simulink model "CSAD_DWC3_linear_4corner"  (R2017a)
settings: Solver=ode5  StartTime=0.0  StopTime=t_sim  FixedStep=0.01  MaxStep=0.01  RelTol=1e-3
values from neighbouring files (symbols this model uses):
  eta_initial = [5; -1; 0]    [Run4corner.m]    (also in Simulation_plot.m = [-4; -2; 0.6*pi])
  nu_initial = [0; 0; 0]    [Run4corner.m]    (also in Simulation_plot.m)
settings Model: Creator=ONLyn  LastModifiedBy=ONLyn

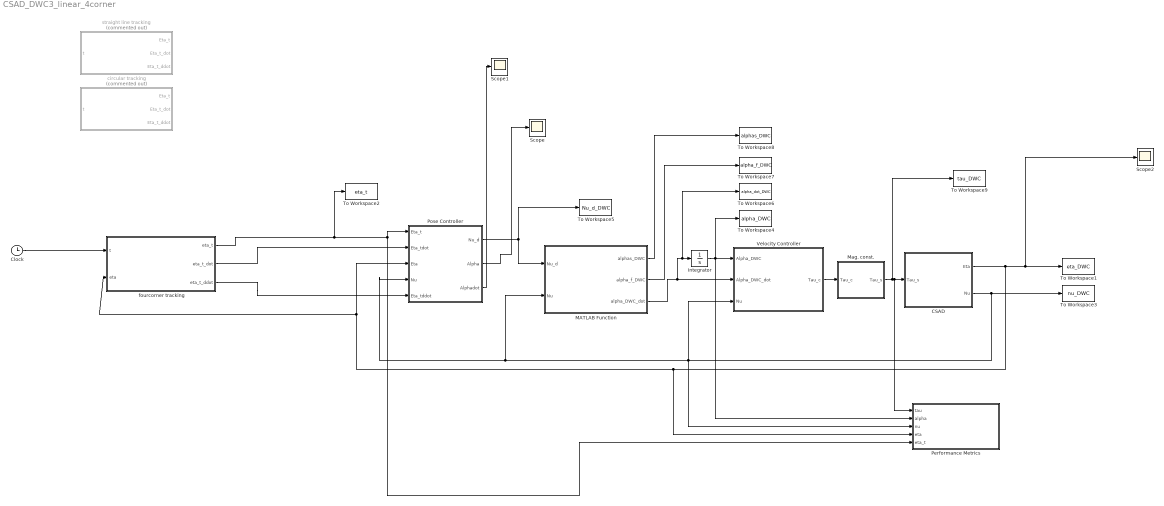
== system CSAD_DWC3_linear_4corner ==
  " Pose Controller" : MATLAB Function  TreatAsAtomicUnit=on
  " Velocity Controller" : MATLAB Function  TreatAsAtomicUnit=on
  " straight line tracking" : MATLAB Function  Commented=on  TreatAsAtomicUnit=on
  CSAD : Subsystem
  Clock : Clock
  Integrator : Integrator  InitialCondition=[0 0 0]
  MATLAB Function : MATLAB Function  TreatAsAtomicUnit=on
  Mag. const. : MATLAB Function  TreatAsAtomicUnit=on
  "Performance Metrics " : Subsystem
  Scope : Scope
  Scope1 : Scope
  Scope2 : Scope
  To Workspace1 : ToWorkspace  VariableName=eta_DWC  SampleTime=-1
  To Workspace2 : ToWorkspace  VariableName=eta_t  SampleTime=-1
  To Workspace3 : ToWorkspace  VariableName=nu_DWC  SampleTime=-1
  To Workspace4 : ToWorkspace  VariableName=alpha_DWC  SampleTime=-1
  To Workspace5 : ToWorkspace  VariableName=Nu_d_DWC  SampleTime=-1
  To Workspace6 : ToWorkspace  VariableName=alpha_dot_DWC  SampleTime=-1
  To Workspace7 : ToWorkspace  VariableName=alpha_f_DWC  SampleTime=-1
  To Workspace8 : ToWorkspace  VariableName=alphas_DWC  SampleTime=-1
  To Workspace9 : ToWorkspace  VariableName=tau_DWC  SampleTime=-1
  circular tracking : MATLAB Function  Commented=on  TreatAsAtomicUnit=on
  fourcorner tracking : Subsystem
  wires:
  CSAD/2(Nu) -> To Workspace3/1, "Performance Metrics "/3(nu), " Velocity Controller"/3(Nu), MATLAB Function/2(Nu), " Pose Controller"/4(Nu)
  CSAD/1(Eta) -> Scope2/1, To Workspace1/1, "Performance Metrics "/4(eta), fourcorner tracking/2(eta), " Pose Controller"/3(Eta)
  " Pose Controller"/1(Nu_d) -> To Workspace5/1, MATLAB Function/1(Nu_d)
  Integrator/1 -> " Velocity Controller"/1(Alpha_DWC), To Workspace4/1, "Performance Metrics "/2(alpha)
  Mag. const./1(Tau_s) -> To Workspace9/1, "Performance Metrics "/1(tau), CSAD/1(Tau_s)
  MATLAB Function/3(alpha_DWC_dot) -> " Velocity Controller"/2(Alpha_DWC_dot), To Workspace6/1, Integrator/1
  MATLAB Function/2(alpha_f_DWC) -> To Workspace7/1
  MATLAB Function/1(alphas_DWC) -> To Workspace8/1
  " Velocity Controller"/1(Tau_c) -> Mag. const./1(Tau_c)
  " Pose Controller"/2(Alpha) -> Scope/1
  " Pose Controller"/3(Alphadot) -> Scope1/1
  fourcorner tracking/1(eta_t) -> "Performance Metrics "/5(eta_t), " Pose Controller"/1(Eta_t), To Workspace2/1
  Clock/1 -> fourcorner tracking/1(t)
  fourcorner tracking/2(eta_t_dot) -> " Pose Controller"/2(Eta_tdot)
  fourcorner tracking/3(eta_t_ddot) -> " Pose Controller"/5(Eta_tddot)

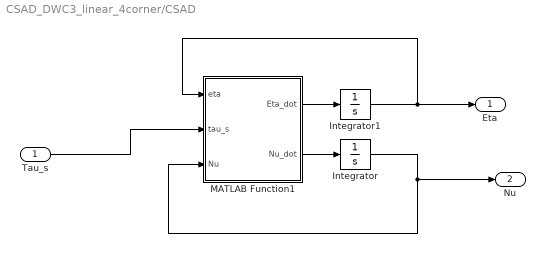
== system CSAD_DWC3_linear_4corner/CSAD ==
  Tau_s : Inport
  Integrator : Integrator  InitialCondition=nu_initial
  Integrator1 : Integrator  InitialCondition=eta_initial
  MATLAB Function1 : MATLAB Function  TreatAsAtomicUnit=on
  Eta : Outport
  Nu : Outport  Port=2
  wires:
  Integrator/1 -> Nu/1, MATLAB Function1/3(Nu)
  MATLAB Function1/1(Eta_dot) -> Integrator1/1
  Integrator1/1 -> Eta/1, MATLAB Function1/1(eta)
  MATLAB Function1/2(Nu_dot) -> Integrator/1
  Tau_s/1 -> MATLAB Function1/2(tau_s)

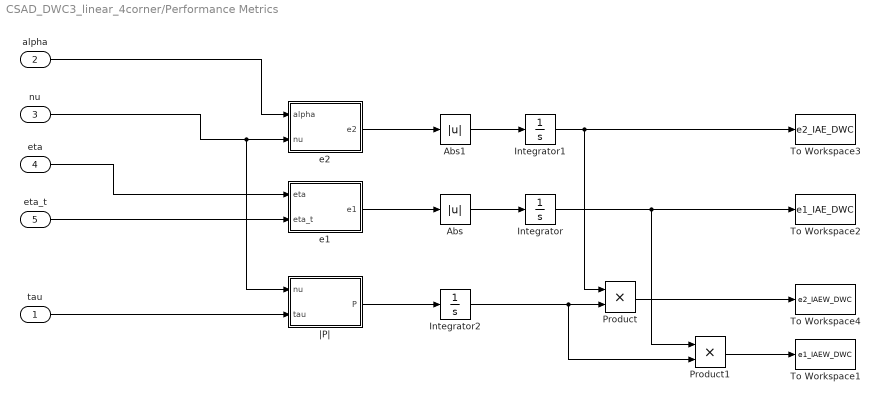
== system CSAD_DWC3_linear_4corner/Performance Metrics  ==
  tau : Inport
  alpha : Inport  Port=2
  nu : Inport  Port=3
  eta : Inport  Port=4
  eta_t : Inport  Port=5
  Abs : Abs
  Abs1 : Abs
  Integrator : Integrator
  Integrator1 : Integrator
  Integrator2 : Integrator
  Product : Product
  Product1 : Product
  To Workspace1 : ToWorkspace  VariableName=e1_IAEW_DWC  SampleTime=-1
  To Workspace2 : ToWorkspace  VariableName=e1_IAE_DWC  SampleTime=-1
  To Workspace3 : ToWorkspace  VariableName=e2_IAE_DWC  SampleTime=-1
  To Workspace4 : ToWorkspace  VariableName=e2_IAEW_DWC  SampleTime=-1
  e1 : MATLAB Function  TreatAsAtomicUnit=on
  "e2 " : MATLAB Function  TreatAsAtomicUnit=on
  |P| : MATLAB Function  TreatAsAtomicUnit=on
  wires:
  Integrator/1 -> Product1/1, To Workspace2/1
  e1/1(e1) -> Abs/1
  "e2 "/1(e2) -> Abs1/1
  Integrator1/1 -> Product/1, To Workspace3/1
  Abs/1 -> Integrator/1
  Abs1/1 -> Integrator1/1
  eta_t/1 -> e1/2(eta_t)
  eta/1 -> e1/1(eta)
  nu/1 -> |P|/1(nu), "e2 "/2(nu)
  alpha/1 -> "e2 "/1(alpha)
  tau/1 -> |P|/2(tau)
  |P|/1(P) -> Integrator2/1
  Integrator2/1 -> Product1/2, Product/2
  Product/1 -> To Workspace4/1
  Product1/1 -> To Workspace1/1

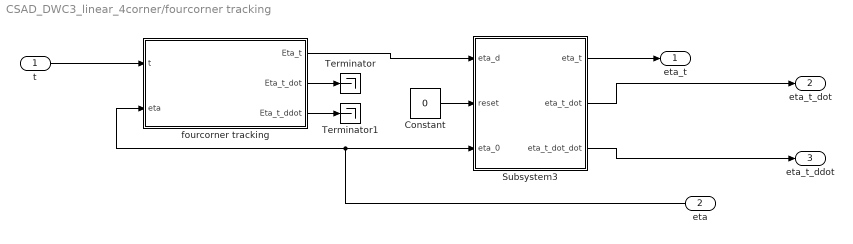
== system CSAD_DWC3_linear_4corner/fourcorner tracking ==
  t : Inport
  eta : Inport  Port=2
  Constant : Constant  Value=0
  Subsystem3 : Subsystem
  Terminator : Terminator
  Terminator1 : Terminator
  fourcorner tracking : MATLAB Function  TreatAsAtomicUnit=on
  eta_t : Outport
  eta_t_dot : Outport  Port=2
  eta_t_ddot : Outport  Port=3
  wires:
  Subsystem3/3(eta_t_dot_dot) -> eta_t_ddot/1
  fourcorner tracking/2(Eta_t_dot) -> Terminator/1
  Constant/1 -> Subsystem3/2(reset)
  Subsystem3/1(eta_t) -> eta_t/1
  t/1 -> fourcorner tracking/1(t)
  eta/1 -> fourcorner tracking/2(eta), Subsystem3/3(eta_0)
  fourcorner tracking/3(Eta_t_ddot) -> Terminator1/1
  fourcorner tracking/1(Eta_t) -> Subsystem3/1(eta_d)
  Subsystem3/2(eta_t_dot) -> eta_t_dot/1

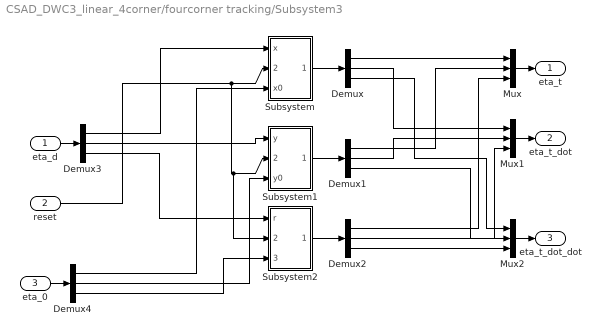
== system CSAD_DWC3_linear_4corner/fourcorner tracking/Subsystem3 ==
  eta_d : Inport
  reset : Inport  Port=2
  eta_0 : Inport  Port=3
  Demux{,1..4} (5 alike) : Demux  Outputs=3
  Mux : Mux  Inputs=3
  Mux1 : Mux  Inputs=3
  Mux2 : Mux  Inputs=3
  Subsystem : Subsystem
  Subsystem1 : Subsystem
  Subsystem2 : Subsystem
  eta_t : Outport  PortDimensions=3
  eta_t_dot : Outport  Port=2  PortDimensions=3
  eta_t_dot_dot : Outport  Port=3  PortDimensions=3
  wires:
  Subsystem1/1(y,yd,ydd) -> Demux1/1
  Subsystem2/1(y,yd,ydd) -> Demux2/1
  Subsystem/1(x,xd,xdd) -> Demux/1
  Demux/3 -> Mux2/1
  eta_d/1 -> Demux3/1
  Mux1/1 -> eta_t_dot/1
  Demux/1 -> Mux/1
  Mux2/1 -> eta_t_dot_dot/1
  Demux3/1 -> Subsystem/1(x)
  Demux1/3 -> Mux2/2
  Demux2/3 -> Mux2/3
  Demux1/1 -> Mux/2
  Demux3/2 -> Subsystem1/1(y)
  Demux3/3 -> Subsystem2/1(r)
  Demux2/2 -> Mux1/3
  Demux1/2 -> Mux1/2
  reset/1 -> Subsystem2/2(reset), Subsystem1/2(reset), Subsystem/2(reset)
  Mux/1 -> eta_t/1
  Demux/2 -> Mux1/1
  Demux2/1 -> Mux/3
  Demux4/3 -> Subsystem2/3(psi0)
  Demux4/2 -> Subsystem1/3(y0)
  Demux4/1 -> Subsystem/3(x0)
  eta_0/1 -> Demux4/1

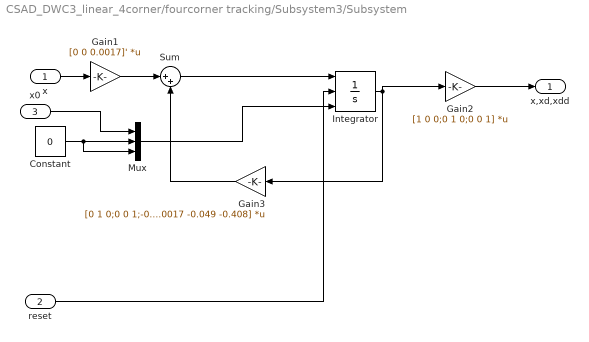
== system CSAD_DWC3_linear_4corner/fourcorner tracking/Subsystem3/Subsystem ==
  x : Inport
  reset : Inport  Port=2
  x0 : Inport  Port=3
  Constant : Constant  Value=0
  Gain1 : Gain  Gain=[0 0 0.0017]'  Multiplication=Matrix(K*u)
  Gain2 : Gain  Gain=[1 0 0;0 1 0;0 0 1]  Multiplication=Matrix(K*u)
  Gain3 : Gain  Gain=[0 1 0;0 0 1;-0.0017 -0.049 -0.408]  Multiplication=Matrix(K*u)
  Integrator : Integrator  ExternalReset=either  InitialConditionSource=external
  Mux : Mux  Inputs=3
  Sum : Sum  Inputs=|++
  x,xd,xdd : Outport  PortDimensions=3
  wires:
  Gain1/1 -> Sum/1
  x/1 -> Gain1/1
  Integrator/1 -> Gain2/1, Gain3/1
  Sum/1 -> Integrator/1
  Gain2/1 -> x,xd,xdd/1
  Mux/1 -> Integrator/3
  reset/1 -> Integrator/2
  Gain3/1 -> Sum/2
  Constant/1 -> Mux/2, Mux/3
  x0/1 -> Mux/1

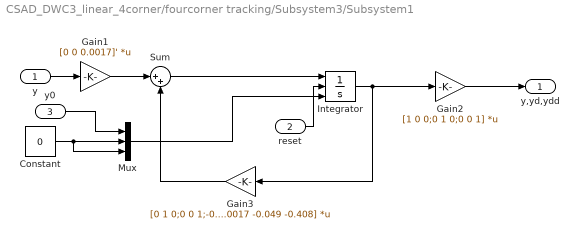
== system CSAD_DWC3_linear_4corner/fourcorner tracking/Subsystem3/Subsystem1 ==
  y : Inport
  reset : Inport  Port=2
  y0 : Inport  Port=3
  Constant : Constant  Value=0
  Gain1 : Gain  Gain=[0 0 0.0017]'  Multiplication=Matrix(K*u)
  Gain2 : Gain  Gain=[1 0 0;0 1 0;0 0 1]  Multiplication=Matrix(K*u)
  Gain3 : Gain  Gain=[0 1 0;0 0 1;-0.0017 -0.049 -0.408]  Multiplication=Matrix(K*u)
  Integrator : Integrator  ExternalReset=either  InitialConditionSource=external
  Mux : Mux  Inputs=3
  Sum : Sum  Inputs=|++
  y,yd,ydd : Outport
  wires:
  Constant/1 -> Mux/3, Mux/2
  Gain3/1 -> Sum/2
  reset/1 -> Integrator/2
  Mux/1 -> Integrator/3
  Gain2/1 -> y,yd,ydd/1
  Sum/1 -> Integrator/1
  Integrator/1 -> Gain3/1, Gain2/1
  y/1 -> Gain1/1
  Gain1/1 -> Sum/1
  y0/1 -> Mux/1

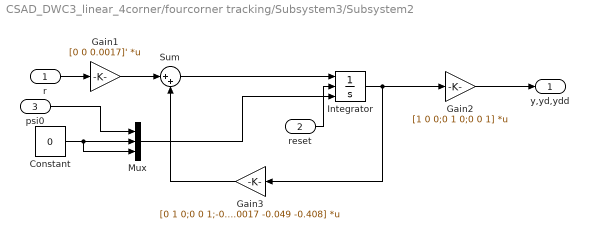
== system CSAD_DWC3_linear_4corner/fourcorner tracking/Subsystem3/Subsystem2 ==
  r : Inport
  reset : Inport  Port=2
  psi0 : Inport  Port=3
  Constant : Constant  Value=0
  Gain1 : Gain  Gain=[0 0 0.0017]'  Multiplication=Matrix(K*u)
  Gain2 : Gain  Gain=[1 0 0;0 1 0;0 0 1]  Multiplication=Matrix(K*u)
  Gain3 : Gain  Gain=[0 1 0;0 0 1;-0.0017 -0.049 -0.408]  Multiplication=Matrix(K*u)
  Integrator : Integrator  ExternalReset=either  InitialConditionSource=external
  Mux : Mux  Inputs=3
  Sum : Sum  Inputs=|++
  y,yd,ydd : Outport
  wires:
  Gain1/1 -> Sum/1
  r/1 -> Gain1/1
  Integrator/1 -> Gain2/1, Gain3/1
  Sum/1 -> Integrator/1
  Gain2/1 -> y,yd,ydd/1
  Mux/1 -> Integrator/3
  reset/1 -> Integrator/2
  Gain3/1 -> Sum/2
  Constant/1 -> Mux/2, Mux/3
  psi0/1 -> Mux/1

== matlab function CSAD_DWC3_linear_4corner/ Velocity Controller ==
  data: Alpha_DWC input; Alpha_DWC_dot input; Tau_c output; Nu input
function Tau_c = VelocityControl(Alpha_DWC, Alpha_DWC_dot,Nu)

[M, C, D] = CSAD_linear2(Nu);

z2 = Nu - Alpha_DWC;

Gamma2 = diag([0.2,0.2 , 0.1745])*M;
delta_v = 0.7;
delta_r = 1;

z2_v = [z2(1), z2(2)]';
z2_r = z2(3);

first = 1/(sqrt(z2_v'*z2_v + delta_v^2));
second = 1/(sqrt(z2_r^2 + delta_r^2));

K2 = Gamma2*[first*eye(2,2) zeros(2,1); zeros(1,2) second];

z2 = Nu - Alpha_DWC;

% full model
% Tau_c = M * Alpha_DWC_dot + C * Alpha_DWC + D * Alpha_DWC;% - K2 * z2;

%linear model
Tau_c = M * Alpha_DWC_dot + D * Alpha_DWC;%-K2 * z2;


end

== matlab function CSAD_DWC3_linear_4corner/MATLAB Function ==
  data: Nu_d input; alphas_DWC output; Nu input; alpha_f_DWC output; alpha_DWC_dot output
function [alphas_DWC, alpha_f_DWC, alpha_DWC_dot] = CSAD_DWC3_linear(Nu_d, Nu)

tau_min = [-1.1089 -0.6387 -0.6176]';
tau_max = [1.1089 0.6387 0.6176]';

% %full model case
% [M,C,D] = CSAD_linear2(Nu);
% Nu_dot_min = inv(M)*(tau_min -C*Nu- D*Nu);
% Nu_dot_max = inv(M)*(tau_max - C*Nu - D*Nu);

% linear model case
[M,C,D] = CSAD_linear2(Nu);
Nu_dot_min = inv(M)*(tau_min - D*Nu);
Nu_dot_max = inv(M)*(tau_max - D*Nu);

ts = 0.05;
Nu_min = Nu+ts*Nu_dot_min;
Nu_max = Nu+ts*Nu_dot_max;

%% Yawrate/surge
u_points_ys = linspace(Nu_min(1),Nu_max(1),7);
r_points_ys = linspace(Nu_min(3),Nu_max(3),7);

if CSAD_g3_linear(Nu_d, 'yawrate_surge')>0 && (Nu_d(1)>= Nu_min(1) && Nu_d(1)<= Nu_max(1)) && (Nu_d(3)>= Nu_min(3) && Nu_d(3)<= Nu_max(3))
    u_diff_ys = u_points_ys-Nu_d(1);
    [~,u_move_ys] = min(abs(u_diff_ys));
    u_points_ys(u_move_ys) = u_points_ys(u_move_ys)-u_diff_ys(u_move_ys);

    r_diff_ys = r_points_ys-Nu_d(3);
    [~,r_move_ys] = min(abs(r_diff_ys));
    r_points_ys(r_move_ys) = r_points_ys(r_move_ys)-r_diff_ys(r_move_ys);
end

if CSAD_g3_linear(Nu_d,'yawrate_surge')>0 && (Nu_d(1)>= Nu_min(1) && Nu_d(1)<= Nu_max(1))
    u_diff_ys = u_points_ys-Nu_d(1);
    [~,u_move_ys] = min(abs(u_diff_ys));
    u_points_ys(u_move_ys) = u_points_ys(u_move_ys)-u_diff_ys(u_move_ys);
end

if CSAD_g3_linear(Nu_d,'yawrate_surge')>0 && (Nu_d(3)>= Nu_min(3) && Nu_d(3)<= Nu_max(3))
    r_diff_ys = r_points_ys-Nu_d(3);
    [~,r_move_ys] = min(abs(r_diff_ys));
    r_points_ys(r_move_ys) = r_points_ys(r_move_ys)-r_diff_ys(r_move_ys);
end

uu_points_ys =[u_points_ys;u_points_ys;u_points_ys;u_points_ys;u_points_ys;u_points_ys;u_points_ys];
rr_points_ys =[r_points_ys;r_points_ys;r_points_ys;r_points_ys;r_points_ys;r_points_ys;r_points_ys]';

uss_ys = reshape(uu_points_ys,[1,49]);
rss_ys = reshape(rr_points_ys,[1,49]);
Nu_r_ys = zeros(3,49);
Nu_r_ys(1,:) = uss_ys;
Nu_r_ys(3,:) = rss_ys;
h = CSAD_g3_linear(Nu_r_ys,'yawrate_surge');

remove_point_ys= find(h>=0);

Nu_f_ys = zeros(3,length(remove_point_ys));
Nu_f_ys(1,:) = uu_points_ys(remove_point_ys);
Nu_f_ys(3,:) = rr_points_ys(remove_point_ys);

Ob_ys = CSAD_objective_function_dw3(Nu_d,Nu_f_ys,'yawrate_surge');

[~,vel_pair_ys] = max(Ob_ys(:,3));

alpha_ys = Nu_f_ys(:,vel_pair_ys);

%% Yawrate/sway
v_points_ysw = linspace(Nu_min(2),Nu_max(2),7);
r_points_ysw = linspace(Nu_min(3),Nu_max(3),7);

if CSAD_g3_linear(Nu_d, 'yawrate_sway')>0 && (Nu_d(2)>= Nu_min(2) && Nu_d(2)<= Nu_max(2)) && (Nu_d(3)>= Nu_min(3) && Nu_d(3)<= Nu_max(3))
    v_diff_ysw = v_points_ysw-Nu_d(2);
    [~,v_move_ysw] = min(abs(v_diff_ysw));
    v_points_ysw(v_move_ysw) = v_points_ysw(v_move_ysw)-v_diff_ysw(v_move_ysw);

    r_diff_ysw = r_points_ysw-Nu_d(3);
    [~,r_move_ysw] = min(abs(r_diff_ysw));
    r_points_ysw(r_move_ysw) = r_points_ysw(r_move_ysw)-r_diff_ysw(r_move_ysw);
end

if CSAD_g3_linear(Nu_d,'yawrate_sway')>0 && (Nu_d(2)>= Nu_min(2) && Nu_d(2)<= Nu_max(2))
    v_diff_ysw = v_points_ysw-Nu_d(2);
    [~,v_move_ysw] = min(abs(v_diff_ysw));
    v_points_ysw(v_move_ysw) = v_points_ysw(v_move_ysw)-v_diff_ysw(v_move_ysw);
end

if CSAD_g3_linear(Nu_d,'yawrate_sway')>0 && (Nu_d(3)>= Nu_min(3) && Nu_d(3)<= Nu_max(3))
    r_diff_ysw = r_points_ysw-Nu_d(3);
    [~,r_move_ysw] = min(abs(r_diff_ysw));
    r_points_ysw(r_move_ysw) = r_points_ysw(r_move_ysw)-r_diff_ysw(r_move_ysw);
end

vv_points_ysw =[v_points_ysw;v_points_ysw;v_points_ysw;v_points_ysw;v_points_ysw;v_points_ysw;v_points_ysw];
rr_points_ysw =[r_points_ysw;r_points_ysw;r_points_ysw;r_points_ysw;r_points_ysw;r_points_ysw;r_points_ysw]';

vss_ysw = reshape(vv_points_ysw,[1,49]);
rss_ysw = reshape(rr_points_ysw,[1,49]);
Nu_r_ysw = zeros(3,49);
Nu_r_ysw(2,:) = vss_ysw;
Nu_r_ysw(3,:) = rss_ysw;
h = CSAD_g3_linear(Nu_r_ysw,'yawrate_sway');

remove_point_ysw= find(h>=0);

Nu_f_ysw = zeros(3,length(remove_point_ysw));
Nu_f_ysw(2,:) = vv_points_ysw(remove_point_ysw);
Nu_f_ysw(3,:) = rr_points_ysw(remove_point_ysw);

Ob_ysw = CSAD_objective_function_dw3(Nu_d,Nu_f_ysw,'yawrate_sway');

[~,vel_pair_ysw] = max(Ob_ysw(:,3));

alpha_ysw = Nu_f_ysw(:,vel_pair_ysw);


%% Sway/Surge
v_points_sws = linspace(Nu_min(2),Nu_max(2),7);
u_points_sws = linspace(Nu_min(1),Nu_max(1),7);

if CSAD_g3_linear(Nu_d, 'sway_surge')>0 && (Nu_d(2)>= Nu_min(2) && Nu_d(2)<= Nu_max(2)) && (Nu_d(1)>= Nu_min(1) && Nu_d(1)<= Nu_max(1))
    v_diff_sws = v_points_sws-Nu_d(2);
    [~,v_move_sws] = min(abs(v_diff_sws));
    v_points_sws(v_move_sws) = v_points_sws(v_move_sws)-v_diff_sws(v_move_sws);

    u_diff_sws = u_points_sws-Nu_d(1);
    [~,u_move_sws] = min(abs(u_diff_sws));
    u_points_sws(u_move_sws) = u_points_sws(u_move_sws)-u_diff_sws(u_move_sws);
end

if CSAD_g3_linear(Nu_d,'sway_surge')>0 && (Nu_d(2)>= Nu_min(2) && Nu_d(2)<= Nu_max(2))
    v_diff_sws = v_points_sws-Nu_d(2);
    [~,v_move_sws] = min(abs(v_diff_sws));
    v_points_sws(v_move_sws) = v_points_sws(v_move_sws)-v_diff_sws(v_move_sws);
end

if CSAD_g3_linear(Nu_d,'sway_surge')>0 && (Nu_d(1)>= Nu_min(1) && Nu_d(1)<= Nu_max(1))
    u_diff_sws = u_points_sws-Nu_d(1);
    [~,u_move_sws] = min(abs(u_diff_sws));
    u_points_sws(u_move_sws) = u_points_sws(u_move_sws)-u_diff_sws(u_move_sws);
end

vv_points_sws =[v_points_sws;v_points_sws;v_points_sws;v_points_sws;v_points_sws;v_points_sws;v_points_sws];
uu_points_sws =[u_points_sws;u_points_sws;u_points_sws;u_points_sws;u_points_sws;u_points_sws;u_points_sws]';

vss_sws = reshape(vv_points_sws,[1,49]);
uss_sws = reshape(uu_points_sws,[1,49]);
Nu_r_sws = zeros(3,49);
Nu_r_sws(2,:) = vss_sws;
Nu_r_sws(1,:) = uss_sws;
h = CSAD_g3_linear(Nu_r_sws,'sway_surge');

remove_point_sws= find(h>=0);

Nu_f_sws = zeros(3,length(remove_point_sws));
Nu_f_sws(2,:) = vv_points_sws(remove_point_sws);
Nu_f_sws(1,:) = uu_points_sws(remove_point_sws);

Ob_sws = CSAD_objective_function_dw3(Nu_d,Nu_f_sws,'sway_surge');

[~,vel_pair_sws] = max(Ob_sws(:,3));

alpha_sws = Nu_f_sws(:,vel_pair_sws);

%% 
alphas_DWC = [alpha_ys,alpha_ysw,alpha_sws];
alpha_f_DWC = (alpha_ys + alpha_ysw + alpha_sws)/2;
alpha_DWC_dot = (alpha_f_DWC - Nu)/ts;

end

== matlab function CSAD_DWC3_linear_4corner/CSAD/MATLAB Function1 ==
  data: eta input; tau_s input; Eta_dot output; Nu input; Nu_dot output
function [Eta_dot,Nu_dot] = Vessel(eta,tau_s,Nu)

Nu_dot = CSAD_full(Nu,tau_s);

yaw = eta(3);

R =[cos(yaw) -sin(yaw) 0;
            sin(yaw)  cos(yaw) 0;
            0         0        1]; 
Eta_dot = R*Nu;
end

== matlab function CSAD_DWC3_linear_4corner/ Pose Controller ==
  data: Eta_t input; Eta_tdot input; Eta input; Nu_d output; Nu input; Alpha output; Alphadot output; Eta_tddot input
function [Nu_d, Alpha ,Alphadot]  = PoseControl(Eta_t, Eta_tdot, Eta, Nu,Eta_tddot)
Gamma1 =  diag([0.08, 0.08, 0.0698]);
delta_psi = 0.5;
delta_p = 0.5;

psi = Eta(3);
r = Nu(3);

S = [0 -r  0; r  0  0; 0  0  0];
S_T = S';
R = [cos(psi) -sin(psi) 0; sin(psi) cos(psi) 0; 0 0 1];
R_T = R';

z1 = R_T * (Eta - Eta_t);

z1_p = [z1(1), z1(2)]';
z1_psi = z1(3);

first = 1/(sqrt(z1_p'*z1_p + delta_p^2));
second = 1/(sqrt(z1_psi^2 + delta_psi^2));

K1 = Gamma1*[first*eye(2,2) zeros(2,1); zeros(1,2) second];

Nu_d = R_T * Eta_tdot - K1 * z1;
Alpha = Nu_d;
z2 = Nu - Alpha;

z1dot = S_T * z1 - K1 * z1 + z2;

z1_p = [z1(1), z1(2)]';
z1_psi = z1(3);
z1_pdot = [z1dot(1), z1dot(2)]';
z1_psidot = z1dot(3);

first2 = (z1_p'*z1_pdot)/((z1_p'*z1_p + delta_p^2)^(3/2));

second2 = (z1_psi*z1_psidot)/((z1_psi^2 + delta_psi^2)^(3/2));

K1dot = - Gamma1*[first2*eye(2,2) zeros(2,1); zeros(1,2) second2];

Alphadot = R_T * Eta_tddot + S_T * R_T * Eta_tdot - K1dot * z1 - K1*z1dot;

end

== matlab function CSAD_DWC3_linear_4corner/Performance Metrics /e1 ==
  data: eta input; e1 output; eta_t input
function e1 = fcn(eta, eta_t)

x = eta(1);
y = eta(2);
psi = eta(3);

x_t = eta_t(1);
y_t = eta_t(2);
psi_t = eta_t(3);

x_tilde = x-x_t;
y_tilde = y-y_t;
psi_tilde = psi-psi_t;

e1 = sqrt(x_tilde^2 + y_tilde^2 + psi_tilde^2);

== matlab function CSAD_DWC3_linear_4corner/Performance Metrics /e2  ==
  data: alpha input; nu input; e2 output
function e2 = fcn(alpha,nu )

u = nu(1);
v = nu(2);
r = nu(3);

u_t = alpha(1);
v_t = alpha(2);
r_t = alpha(3);

u_tilde = u-u_t;
v_tilde = v-v_t;
r_tilde = r-r_t;

e2 = sqrt(u_tilde^2 + v_tilde^2 + r_tilde^2);

== matlab function CSAD_DWC3_linear_4corner/Performance Metrics /|P| ==
  data: nu input; P output; tau input
function P  = fcn(nu, tau)

P = abs(nu' * tau);

== matlab function CSAD_DWC3_linear_4corner/ straight line tracking ==
  data: Eta_t output; Eta_t_dot output; Eta_t_ddot output; t input
function [Eta_t, Eta_t_dot, Eta_t_ddot]   = straightline_tracking(t)

%initial values for track
v_t = 0.15; %m/s
%v_t_dot = 0;

psi_t = 0.9273; %rad
psi_t_dot = 0; %rad/s

x_t = 1 + v_t*t*cos(psi_t);
x_t_dot = v_t*cos(psi_t);
%x_t_ddot = 0;

y_t = v_t*t*sin(psi_t);
y_t_dot = v_t*sin(psi_t);
%y_t_ddot = 0;

if t == 0
    Eta_t = [1; 0; psi_t]; %m m rad
    Eta_t_dot = [0.09; 0.12; 0]; %m/s m/s rad/s
    Eta_t_ddot = [0; 0; 0];
else
    Eta_t = [x_t; y_t; psi_t];
    Eta_t_dot = [x_t_dot; y_t_dot; psi_t_dot];
    Eta_t_ddot = [0; 0; 0];
end


end

== matlab function CSAD_DWC3_linear_4corner/circular tracking ==
  data: Eta_t output; t input; Eta_t_dot output; Eta_t_ddot output
function [Eta_t, Eta_t_dot, Eta_t_ddot] = circular_tracking(t)

r_c = 5;
v_t= 0.15;

x_t = r_c*cos(v_t*t/r_c);
x_t_dot = -v_t*sin(v_t*t/r_c);
x_t_ddot = -(v_t^2)/(r_c)*cos(v_t*t/r_c);
 
y_t = r_c*sin(v_t*t/r_c);
y_t_dot = v_t*cos(v_t*t/r_c);
y_t_ddot = -(v_t^2)/(r_c)*sin(v_t*t/r_c);

tend = 1/(v_t/r_c)*2*pi;
psi_t = 2*pi/tend*t+pi/2;
psi_t_dot = 2*pi/tend;

if t == 0
    Eta_t = [5; 0; 1.5708]; %m m rad
    Eta_t_dot = [0;0;0];
    Eta_t_ddot = [0;0;0];
else
    Eta_t = [x_t; y_t; psi_t];
    Eta_t_dot = [x_t_dot; y_t_dot; psi_t_dot];
    Eta_t_ddot = [x_t_ddot; y_t_ddot; 0];
end
end

== matlab function CSAD_DWC3_linear_4corner/Mag. const. ==
  data: Tau_c input; Tau_s output
function Tau_s = saturatioin(Tau_c)

mag_constr = [1.1089 0.6387 0.6176]'; %N
Tau_s = [0;0;0];

for n = 1:length(Tau_c)
    
    if Tau_c(n) <= -mag_constr(n)
        Tau_s(n) = -mag_constr(n);
    end
    
    if ((Tau_c(n) > -mag_constr(n)) && (Tau_c(n) < mag_constr(n)))
        Tau_s(n) = Tau_c(n);
    end
    
    if Tau_c(n) >= mag_constr(n)
        Tau_s(n) = mag_constr(n);
    end
    
end
    
end

== matlab function CSAD_DWC3_linear_4corner/fourcorner tracking/fourcorner tracking ==
  data: t input; Eta_t output; Eta_t_dot output; Eta_t_ddot output; eta input
function [ Eta_t, Eta_t_dot, Eta_t_ddot]   =  fourcorner_tracking(t,eta)

v_t = 0.15;

etaP = [5 7 7 7 5 5;
       -1 -1 1 1 1 -1;
        0 0 0 pi/4 pi/4 0];
Eta_t_dot = [0;0;0];
Eta_t_ddot = [0;0;0];

Eta_t = [5;-1;0];
persistent point ;
if(isempty(point))
    point = 1;
    
end



switch point
    case 1
        Eta_t = etaP(:,2);
         if ((abs((Eta_t(1)- eta(1))) <0.01 ) ==1  ) && ((abs(Eta_t(2)-eta(2))<0.01) ==1) && (abs(Eta_t(3)-rad2deg(eta(3)))<3 == 1)
            point = 2;
            return;
         end
        
        
    case 2
        Eta_t = etaP(:,3);
        if((abs((Eta_t(1)- eta(1))) <0.01 ) ==1  ) && ((abs(Eta_t(2)-eta(2))<0.01) ==1) && (abs(Eta_t(3)-rad2deg(eta(3)))<3 == 1) 
            point = 3;
            return;
         end
    case 3
        Eta_t = etaP(:,4);
        if((abs((Eta_t(1)- eta(1))) <0.01 ) ==1  ) && ((abs(Eta_t(2)-eta(2))<0.01) ==1) && (rad2deg(abs(Eta_t(3)-eta(3)))<3 == 1)  
            point = 4;
            return;
            
         end
    case 4
        Eta_t = etaP(:,5);
        if((abs((Eta_t(1)- eta(1))) <0.01 ) ==1  ) && ((abs(Eta_t(2)-eta(2))<0.01) ==1) && (rad2deg(abs(Eta_t(3)-eta(3)))<3 == 1) 
            point = 5; 
            return;
         end
    case 5
        Eta_t = etaP(:,6);
        if((abs((Eta_t(1)- eta(1))) <0.01 ) ==1  ) && ((abs(Eta_t(2)-eta(2))<0.01) ==1) && (abs(Eta_t(3)-rad2deg(eta(3)))<3 == 1) 
            point = 6; 
            return;
         end

    otherwise
        

end
end
%(abs(Eta_t(2)-eta(2))<0.01) &&
